simulink model "D53_LKAS_JLU_20200908_1055"  (R2018b)
settings: Solver=ode3  StartTime=0.0  StopTime=10.0  FixedStep=0.01  RelTol=1e-3  EnableMultiTasking=on
model workspace (MAT data in the model file):
  LKA_CarWidth = Simulink.Parameter
  LKA_CarWidth.Value = 1.8
  LKA_CarWidth.DataType = 'single'
  LKA_CarWidth.Dimensions = [1 1]
  LKA_SampleTime = Simulink.Parameter
  LKA_SampleTime.Value = 0.01
  LKA_SampleTime.DataType = 'single'
  LKA_SampleTime.Dimensions = [1 1]
  LKA_StrRatio_C = Simulink.Parameter
  LKA_StrRatio_C.Value = 15.3
  LKA_StrRatio_C.DataType = 'single'
  LKA_StrRatio_C.Dimensions = [1 1]
  LKA_Veh2CamL_C = Simulink.Parameter
  LKA_Veh2CamL_C.Value = 1.56
  LKA_Veh2CamL_C.DataType = 'single'
  LKA_Veh2CamL_C.Dimensions = [1 1]
  LKA_Veh2CamW_C = Simulink.Parameter
  LKA_Veh2CamW_C.Value = 0.9
  LKA_Veh2CamW_C.DataType = 'single'
  LKA_Veh2CamW_C.Dimensions = [1 1]
  LKA_WhlBaseL_C = Simulink.Parameter
  LKA_WhlBaseL_C.Value = 2.65
  LKA_WhlBaseL_C.DataType = 'single'
  LKA_WhlBaseL_C.Dimensions = [1 1]
  LL_CompSWA_C = Simulink.Parameter
  LL_CompSWA_C.Value = 0
  LL_CompSWA_C.DataType = 'single'
  LL_CompSWA_C.Dimensions = [1 1]
  LL_CrvtPrvwT_C = Simulink.Parameter
  LL_CrvtPrvwT_C.Value = 0.45
  LL_CrvtPrvwT_C.DataType = 'single'
  LL_CrvtPrvwT_C.Dimensions = [1 1]
  LL_DesDvt_C = Simulink.Parameter
  LL_DesDvt_C.Value = 0.2
  LL_DesDvt_C.DataType = 'single'
  LL_DesDvt_C.Dimensions = [1 1]
  LL_DvtComp_C = Simulink.Parameter
  LL_DvtComp_C.Value = 0
  LL_DvtComp_C.DataType = 'single'
  LL_DvtComp_C.Dimensions = [1 1]
  LL_DvtPrvwT_C = Simulink.Parameter
  LL_DvtPrvwT_C.Value = 0.45
  LL_DvtPrvwT_C.DataType = 'single'
  LL_DvtPrvwT_C.Dimensions = [1 1]
  LL_DvtSpdDet_vDvtSpdMin_C = Simulink.Parameter
  LL_DvtSpdDet_vDvtSpdMin_C.Value = 0
  LL_DvtSpdDet_vDvtSpdMin_C.DataType = 'single'
  LL_DvtSpdDet_vDvtSpdMin_C.Dimensions = [1 1]
  LL_HdAgExT_C = Simulink.Parameter
  LL_HdAgExT_C.Value = 15
  LL_HdAgExT_C.DataType = 'single'
  LL_HdAgExT_C.Dimensions = [1 1]
  LL_HdAgPrvwT_C = Simulink.Parameter
  LL_HdAgPrvwT_C.Value = 0.45
  LL_HdAgPrvwT_C.DataType = 'single'
  LL_HdAgPrvwT_C.Dimensions = [1 1]
  LL_LAccMax_C = Simulink.Parameter
  LL_LAccMax_C.Value = 3
  LL_LAccMax_C.DataType = 'single'
  LL_LAccMax_C.Dimensions = [1 1]
  LL_LAccRMax_C = Simulink.Parameter
  LL_LAccRMax_C.Value = 5
  LL_LAccRMax_C.DataType = 'single'
  LL_LAccRMax_C.Dimensions = [1 1]
  LL_LDWS_SUPPRESS_HEADING = Simulink.Parameter
  LL_LDWS_SUPPRESS_HEADING.Value = 2
  LL_LDWS_SUPPRESS_HEADING.DataType = 'single'
  LL_LDWS_SUPPRESS_HEADING.Dimensions = [1 1]
  LL_LDW_EarliestWarnLine_C = Simulink.Parameter
  LL_LDW_EarliestWarnLine_C.Value = 0.3
  LL_LDW_EarliestWarnLine_C.DataType = 'single'
  LL_LDW_EarliestWarnLine_C.Dimensions = [1 1]
  LL_LDW_LatestWarnLine_C = Simulink.Parameter
  LL_LDW_LatestWarnLine_C.Value = -0.4
  LL_LDW_LatestWarnLine_C.DataType = 'single'
  LL_LDW_LatestWarnLine_C.Dimensions = [1 1]
  LL_LFClb_TFC_DiffCtlBalance = Simulink.Parameter
  LL_LFClb_TFC_DiffCtlBalance.Value = 0
  LL_LFClb_TFC_DiffCtlBalance.DataType = 'single'
  LL_LFClb_TFC_DiffCtlBalance.Dimensions = [1 1]
  LL_LFClb_TFC_DiffCtrlMaxSWA = Simulink.Parameter
  LL_LFClb_TFC_DiffCtrlMaxSWA.Value = 20
  LL_LFClb_TFC_DiffCtrlMaxSWA.DataType = 'single'
  LL_LFClb_TFC_DiffCtrlMaxSWA.Dimensions = [1 1]
  LL_LFClb_TFC_DiffCtrlRatio = Simulink.Parameter
  LL_LFClb_TFC_DiffCtrlRatio.Value = 400
  LL_LFClb_TFC_DiffCtrlRatio.DataType = 'single'
  LL_LFClb_TFC_DiffCtrlRatio.Dimensions = [1 1]
  LL_LFClb_TFC_FfCtlRatio_C = Simulink.Parameter
  LL_LFClb_TFC_FfCtlRatio_C.Value = 1
  LL_LFClb_TFC_FfCtlRatio_C.DataType = 'single'
  LL_LFClb_TFC_FfCtlRatio_C.Dimensions = [1 1]
  LL_LFClb_TFC_facmGainLutGain1_C = Simulink.Parameter
  LL_LFClb_TFC_facmGainLutGain1_C.Value = 40
  LL_LFClb_TFC_facmGainLutGain1_C.DataType = 'single'
  LL_LFClb_TFC_facmGainLutGain1_C.Dimensions = [1 1]
  LL_LFClb_TFC_facmGainLutGain2_C = Simulink.Parameter
  LL_LFClb_TFC_facmGainLutGain2_C.Value = 40
  LL_LFClb_TFC_facmGainLutGain2_C.DataType = 'single'
  LL_LFClb_TFC_facmGainLutGain2_C.Dimensions = [1 1]
  LL_LFClb_TFC_facmIntegRatio = Simulink.Parameter
  LL_LFClb_TFC_facmIntegRatio.Value = 0.002
  LL_LFClb_TFC_facmIntegRatio.DataType = 'single'
  LL_LFClb_TFC_facmIntegRatio.Dimensions = [1 1]
  LL_LFClb_TFC_facmKlat_C = Simulink.Parameter
  LL_LFClb_TFC_facmKlat_C.Value = -9
  LL_LFClb_TFC_facmKlat_C.DataType = 'single'
  LL_LFClb_TFC_facmKlat_C.Dimensions = [1 1]
  LL_LFClb_TFC_phiIntegCtlMaxSWA_C = Simulink.Parameter
  LL_LFClb_TFC_phiIntegCtlMaxSWA_C.Value = 5
  LL_LFClb_TFC_phiIntegCtlMaxSWA_C.DataType = 'single'
  LL_LFClb_TFC_phiIntegCtlMaxSWA_C.Dimensions = [1 1]
  LL_LFClb_TFC_tiKlatPrvwT_C = Simulink.Parameter
  LL_LFClb_TFC_tiKlatPrvwT_C.Value = 2
  LL_LFClb_TFC_tiKlatPrvwT_C.DataType = 'single'
  LL_LFClb_TFC_tiKlatPrvwT_C.Dimensions = [1 1]
  LL_LFClb_TFC_vGainLutVehSpdLwr_C = Simulink.Parameter
  LL_LFClb_TFC_vGainLutVehSpdLwr_C.Value = 60
  LL_LFClb_TFC_vGainLutVehSpdLwr_C.DataType = 'single'
  LL_LFClb_TFC_vGainLutVehSpdLwr_C.Dimensions = [1 1]
  LL_LFClb_TFC_vGainLutVehSpdUpr_C = Simulink.Parameter
  LL_LFClb_TFC_vGainLutVehSpdUpr_C.Value = 120
  LL_LFClb_TFC_vGainLutVehSpdUpr_C.DataType = 'single'
  LL_LFClb_TFC_vGainLutVehSpdUpr_C.Dimensions = [1 1]
  LL_LKAExPrcs_ExitC0Dvt = Simulink.Parameter
  LL_LKAExPrcs_ExitC0Dvt.Value = 0.01
  LL_LKAExPrcs_ExitC0Dvt.DataType = 'single'
  LL_LKAExPrcs_ExitC0Dvt.Dimensions = [1 1]
  LL_LKAExPrcs_ExitC0Swt = Simulink.Parameter
  LL_LKAExPrcs_ExitC0Swt.Value = 1
  LL_LKAExPrcs_ExitC0Swt.DataType = 'single'
  LL_LKAExPrcs_ExitC0Swt.Dimensions = [1 1]
  LL_LKAExPrcs_tiExitTime1 = Simulink.Parameter
  LL_LKAExPrcs_tiExitTime1.Value = 8
  LL_LKAExPrcs_tiExitTime1.DataType = 'single'
  LL_LKAExPrcs_tiExitTime1.Dimensions = [1 1]
  LL_LKAExPrcs_tiExitTime2 = Simulink.Parameter
  LL_LKAExPrcs_tiExitTime2.Value = 4
  LL_LKAExPrcs_tiExitTime2.DataType = 'single'
  LL_LKAExPrcs_tiExitTime2.Dimensions = [1 1]
  LL_LKAExPrcs_tiExitTime3 = Simulink.Parameter
  LL_LKAExPrcs_tiExitTime3.Value = 0.2
  LL_LKAExPrcs_tiExitTime3.DataType = 'single'
  LL_LKAExPrcs_tiExitTime3.Dimensions = [1 1]
  LL_LKASWASyn_M0 = Simulink.Parameter
  LL_LKASWASyn_M0.Value = 0.4
  LL_LKASWASyn_M0.DataType = 'single'
  LL_LKASWASyn_M0.Dimensions = [1 1]
  LL_LKASWASyn_M1 = Simulink.Parameter
  LL_LKASWASyn_M1.Value = 0.8
  LL_LKASWASyn_M1.DataType = 'single'
  LL_LKASWASyn_M1.Dimensions = [1 1]
  LL_LKASWASyn_M2 = Simulink.Parameter
  LL_LKASWASyn_M2.Value = 0.3
  LL_LKASWASyn_M2.DataType = 'single'
  LL_LKASWASyn_M2.Dimensions = [1 1]
  LL_LKASWASyn_M3K = Simulink.Parameter
  LL_LKASWASyn_M3K.Value = 0.2
  LL_LKASWASyn_M3K.DataType = 'single'
  LL_LKASWASyn_M3K.Dimensions = [1 1]
  LL_LKASWASyn_SWAaddMax = Simulink.Parameter
  LL_LKASWASyn_SWAaddMax.Value = 8
  LL_LKASWASyn_SWAaddMax.DataType = 'single'
  LL_LKASWASyn_SWAaddMax.Dimensions = [1 1]
  LL_LKASWASyn_T2 = Simulink.Parameter
  LL_LKASWASyn_T2.Value = 4
  LL_LKASWASyn_T2.DataType = 'single'
  LL_LKASWASyn_T2.Dimensions = [1 1]
  LL_LKASWASyn_TrqMax = Simulink.Parameter
  LL_LKASWASyn_TrqMax.Value = 1.5
  LL_LKASWASyn_TrqMax.DataType = 'single'
  LL_LKASWASyn_TrqMax.Dimensions = [1 1]
  LL_LKASWASyn_TrqSwaAddSwt = Simulink.Parameter
  LL_LKASWASyn_TrqSwaAddSwt.Value = 0
  LL_LKASWASyn_TrqSwaAddSwt.DataType = 'single'
  LL_LKASWASyn_TrqSwaAddSwt.Dimensions = [1 1]
  LL_LKASWASyn_TrqSwaRateDiff = Simulink.Parameter
  LL_LKASWASyn_TrqSwaRateDiff.Value = -0.2
  LL_LKASWASyn_TrqSwaRateDiff.DataType = 'single'
  LL_LKASWASyn_TrqSwaRateDiff.Dimensions = [1 1]
  LL_LKASWASyn_tiTrqSwaRtTime = Simulink.Parameter
  LL_LKASWASyn_tiTrqSwaRtTime.Value = 0.2
  LL_LKASWASyn_tiTrqSwaRtTime.DataType = 'single'
  LL_LKASWASyn_tiTrqSwaRtTime.Dimensions = [1 1]
  LL_LKASWASyn_tiTrqSwaTime = Simulink.Parameter
  LL_LKASWASyn_tiTrqSwaTime.Value = 0.3
  LL_LKASWASyn_tiTrqSwaTime.DataType = 'single'
  LL_LKASWASyn_tiTrqSwaTime.Dimensions = [1 1]
  LL_LKAS_OUT_OF_CONTROL_LAT_VEL = Simulink.Parameter
  LL_LKAS_OUT_OF_CONTROL_LAT_VEL.Value = 1.5
  LL_LKAS_OUT_OF_CONTROL_LAT_VEL.DataType = 'single'
  LL_LKAS_OUT_OF_CONTROL_LAT_VEL.Dimensions = [1 1]
  LL_LKAS_OUT_OF_CONTROL_TTLC = Simulink.Parameter
  LL_LKAS_OUT_OF_CONTROL_TTLC.Value = 0.3
  LL_LKAS_OUT_OF_CONTROL_TTLC.DataType = 'single'
  LL_LKAS_OUT_OF_CONTROL_TTLC.Dimensions = [1 1]
  LL_LKA_EarliestWarnLine_C = Simulink.Parameter
  LL_LKA_EarliestWarnLine_C.Value = 0.3
  LL_LKA_EarliestWarnLine_C.DataType = 'single'
  LL_LKA_EarliestWarnLine_C.Dimensions = [1 1]
  LL_LKA_LatestWarnLine_C = Simulink.Parameter
  LL_LKA_LatestWarnLine_C.Value = -0.5
  LL_LKA_LatestWarnLine_C.DataType = 'single'
  LL_LKA_LatestWarnLine_C.Dimensions = [1 1]
  LL_LSpdCompT_C = Simulink.Parameter
  LL_LSpdCompT_C.Value = 0.4
  LL_LSpdCompT_C.DataType = 'single'
  LL_LSpdCompT_C.Dimensions = [1 1]
  LL_MAX_DELAY_EPSSTAR_TIME = Simulink.Parameter
  LL_MAX_DELAY_EPSSTAR_TIME.Value = 0.5
  LL_MAX_DELAY_EPSSTAR_TIME.DataType = 'single'
  LL_MAX_DELAY_EPSSTAR_TIME.Dimensions = [1 1]
  LL_MAX_DRIVER_TORQUE_DISABLE = Simulink.Parameter
  LL_MAX_DRIVER_TORQUE_DISABLE.Value = 2.25
  LL_MAX_DRIVER_TORQUE_DISABLE.DataType = 'single'
  LL_MAX_DRIVER_TORQUE_DISABLE.Dimensions = [1 1]
  LL_MAX_DRIVER_TORQUE_ENABLE = Simulink.Parameter
  LL_MAX_DRIVER_TORQUE_ENABLE.Value = 3
  LL_MAX_DRIVER_TORQUE_ENABLE.DataType = 'single'
  LL_MAX_DRIVER_TORQUE_ENABLE.Dimensions = [1 1]
  LL_MAX_LANE_WIDTH_DISABLE = Simulink.Parameter
  LL_MAX_LANE_WIDTH_DISABLE.Value = 5.5
  LL_MAX_LANE_WIDTH_DISABLE.DataType = 'single'
  LL_MAX_LANE_WIDTH_DISABLE.Dimensions = [1 1]
  LL_MAX_LANE_WIDTH_ENABLE = Simulink.Parameter
  LL_MAX_LANE_WIDTH_ENABLE.Value = 5.4
  LL_MAX_LANE_WIDTH_ENABLE.DataType = 'single'
  LL_MAX_LANE_WIDTH_ENABLE.Dimensions = [1 1]
  LL_MAX_LAT_ACC_DISABLE = Simulink.Parameter
  LL_MAX_LAT_ACC_DISABLE.Value = 3.5
  LL_MAX_LAT_ACC_DISABLE.DataType = 'single'
  LL_MAX_LAT_ACC_DISABLE.Dimensions = [1 1]
  LL_MAX_LAT_ACC_ENABLE = Simulink.Parameter
  LL_MAX_LAT_ACC_ENABLE.Value = 3
  LL_MAX_LAT_ACC_ENABLE.DataType = 'single'
  LL_MAX_LAT_ACC_ENABLE.Dimensions = [1 1]
  LL_MAX_LDWS_SPEED_DISABLE = Simulink.Parameter
  LL_MAX_LDWS_SPEED_DISABLE.Value = 150
  LL_MAX_LDWS_SPEED_DISABLE.DataType = 'single'
  LL_MAX_LDWS_SPEED_DISABLE.Dimensions = [1 1]
  LL_MAX_LDWS_SPEED_ENABLE = Simulink.Parameter
  LL_MAX_LDWS_SPEED_ENABLE.Value = 140
  LL_MAX_LDWS_SPEED_ENABLE.DataType = 'single'
  LL_MAX_LDWS_SPEED_ENABLE.Dimensions = [1 1]
  LL_MAX_LKAS_SPEED_DISABLE = Simulink.Parameter
  LL_MAX_LKAS_SPEED_DISABLE.Value = 150
  LL_MAX_LKAS_SPEED_DISABLE.DataType = 'single'
  LL_MAX_LKAS_SPEED_DISABLE.Dimensions = [1 1]
  LL_MAX_LKAS_SPEED_ENABLE = Simulink.Parameter
  LL_MAX_LKAS_SPEED_ENABLE.Value = 140
  LL_MAX_LKAS_SPEED_ENABLE.DataType = 'single'
  LL_MAX_LKAS_SPEED_ENABLE.Dimensions = [1 1]
  LL_MAX_LONG_ACC_DISABLE = Simulink.Parameter
  LL_MAX_LONG_ACC_DISABLE.Value = 3.5
  LL_MAX_LONG_ACC_DISABLE.DataType = 'single'
  LL_MAX_LONG_ACC_DISABLE.Dimensions = [1 1]
  LL_MAX_LONG_ACC_ENABLE = Simulink.Parameter
  LL_MAX_LONG_ACC_ENABLE.Value = 3
  LL_MAX_LONG_ACC_ENABLE.DataType = 'single'
  LL_MAX_LONG_ACC_ENABLE.Dimensions = [1 1]
  LL_MAX_LONG_DECEL_DISABLE = Simulink.Parameter
  LL_MAX_LONG_DECEL_DISABLE.Value = 2.5
  LL_MAX_LONG_DECEL_DISABLE.DataType = 'single'
  LL_MAX_LONG_DECEL_DISABLE.Dimensions = [1 1]
  LL_MAX_LONG_DECEL_ENABLE = Simulink.Parameter
  LL_MAX_LONG_DECEL_ENABLE.Value = 2
  LL_MAX_LONG_DECEL_ENABLE.DataType = 'single'
  LL_MAX_LONG_DECEL_ENABLE.Dimensions = [1 1]
  LL_MAX_STEER_ANGLE_DISABLE = Simulink.Parameter
  LL_MAX_STEER_ANGLE_DISABLE.Value = 70
  LL_MAX_STEER_ANGLE_DISABLE.DataType = 'single'
  LL_MAX_STEER_ANGLE_DISABLE.Dimensions = [1 1]
  LL_MAX_STEER_ANGLE_ENABLE = Simulink.Parameter
  LL_MAX_STEER_ANGLE_ENABLE.Value = 60
  LL_MAX_STEER_ANGLE_ENABLE.DataType = 'single'
  LL_MAX_STEER_ANGLE_ENABLE.Dimensions = [1 1]
  LL_MAX_STEER_SPEED_DISABLE = Simulink.Parameter
  LL_MAX_STEER_SPEED_DISABLE.Value = 5000
  LL_MAX_STEER_SPEED_DISABLE.DataType = 'single'
  LL_MAX_STEER_SPEED_DISABLE.Dimensions = [1 1]
  LL_MAX_STEER_SPEED_ENABLE = Simulink.Parameter
  LL_MAX_STEER_SPEED_ENABLE.Value = 5000
  LL_MAX_STEER_SPEED_ENABLE.DataType = 'single'
  LL_MAX_STEER_SPEED_ENABLE.Dimensions = [1 1]
  LL_MAX_SYSTEM_CURVATURE_DISABLE = Simulink.Parameter
  LL_MAX_SYSTEM_CURVATURE_DISABLE.Value = 0.0055
  LL_MAX_SYSTEM_CURVATURE_DISABLE.DataType = 'single'
  LL_MAX_SYSTEM_CURVATURE_DISABLE.Dimensions = [1 1]
  LL_MAX_SYSTEM_CURVATURE_ENABLE = Simulink.Parameter
  LL_MAX_SYSTEM_CURVATURE_ENABLE.Value = 0.0045
  LL_MAX_SYSTEM_CURVATURE_ENABLE.DataType = 'single'
  LL_MAX_SYSTEM_CURVATURE_ENABLE.Dimensions = [1 1]
  LL_MIN_LANE_WIDTH_DISABLE = Simulink.Parameter
  LL_MIN_LANE_WIDTH_DISABLE.Value = 2.4
  LL_MIN_LANE_WIDTH_DISABLE.DataType = 'single'
  LL_MIN_LANE_WIDTH_DISABLE.Dimensions = [1 1]
  LL_MIN_LANE_WIDTH_ENABLE = Simulink.Parameter
  LL_MIN_LANE_WIDTH_ENABLE.Value = 2.5
  LL_MIN_LANE_WIDTH_ENABLE.DataType = 'single'
  LL_MIN_LANE_WIDTH_ENABLE.Dimensions = [1 1]
  LL_MIN_LKAS_SPEED_DISABLE = Simulink.Parameter
  LL_MIN_LKAS_SPEED_DISABLE.Value = 55
  LL_MIN_LKAS_SPEED_DISABLE.DataType = 'single'
  LL_MIN_LKAS_SPEED_DISABLE.Dimensions = [1 1]
  LL_MIN_LKAS_SPEED_ENABLE = Simulink.Parameter
  LL_MIN_LKAS_SPEED_ENABLE.Value = 60
  LL_MIN_LKAS_SPEED_ENABLE.DataType = 'single'
  LL_MIN_LKAS_SPEED_ENABLE.Dimensions = [1 1]
  LL_Max_LDWS_Warning_Time = Simulink.Parameter
  LL_Max_LDWS_Warning_Time.Value = 5
  LL_Max_LDWS_Warning_Time.DataType = 'single'
  LL_Max_LDWS_Warning_Time.Dimensions = [1 1]
  LL_NomTAhd_C = Simulink.Parameter
  LL_NomTAhd_C.Value = 0.2
  LL_NomTAhd_C.DataType = 'single'
  LL_NomTAhd_C.Dimensions = [1 1]
  LL_ThresDet_lDvtThresLwrLDW = Simulink.Parameter
  LL_ThresDet_lDvtThresLwrLDW.Value = 0.15
  LL_ThresDet_lDvtThresLwrLDW.DataType = 'single'
  LL_ThresDet_lDvtThresLwrLDW.Dimensions = [1 1]
  LL_ThresDet_lDvtThresLwrLKA = Simulink.Parameter
  LL_ThresDet_lDvtThresLwrLKA.Value = 0.3
  LL_ThresDet_lDvtThresLwrLKA.DataType = 'single'
  LL_ThresDet_lDvtThresLwrLKA.Dimensions = [1 1]
  LL_ThresDet_lDvtThresUprLDW = Simulink.Parameter
  LL_ThresDet_lDvtThresUprLDW.Value = 0.3
  LL_ThresDet_lDvtThresUprLDW.DataType = 'single'
  LL_ThresDet_lDvtThresUprLDW.Dimensions = [1 1]
  LL_ThresDet_lDvtThresUprLKA = Simulink.Parameter
  LL_ThresDet_lDvtThresUprLKA.Value = 0.6
  LL_ThresDet_lDvtThresUprLKA.DataType = 'single'
  LL_ThresDet_lDvtThresUprLKA.Dimensions = [1 1]
  LL_ThresDet_tiTTLCThresLDW = Simulink.Parameter
  LL_ThresDet_tiTTLCThresLDW.Value = 0.75
  LL_ThresDet_tiTTLCThresLDW.DataType = 'single'
  LL_ThresDet_tiTTLCThresLDW.Dimensions = [1 1]
  LL_ThresDet_tiTTLCThresLKA = Simulink.Parameter
  LL_ThresDet_tiTTLCThresLKA.Value = 1.5
  LL_ThresDet_tiTTLCThresLKA.DataType = 'single'
  LL_ThresDet_tiTTLCThresLKA.Dimensions = [1 1]
  LL_TkOvStChk_tiTDelTime = Simulink.Parameter
  LL_TkOvStChk_tiTDelTime.Value = 2
  LL_TkOvStChk_tiTDelTime.DataType = 'single'
  LL_TkOvStChk_tiTDelTime.Dimensions = [1 1]
  LL_TkOvStChk_tiTrqChkT = Simulink.Parameter
  LL_TkOvStChk_tiTrqChkT.Value = 0.1
  LL_TkOvStChk_tiTrqChkT.DataType = 'single'
  LL_TkOvStChk_tiTrqChkT.Dimensions = [1 1]
  LL_lStpLngth_C = Simulink.Parameter
  LL_lStpLngth_C.Value = 5
  LL_lStpLngth_C.DataType = 'single'
  LL_lStpLngth_C.Dimensions = [1 1]
  ob_LKA_Version = Simulink.Signal
  ob_LKA_Version.DataType = 'single'
  ob_LKA_Version.Dimensions = -1
  ob_LKA_Version.DimensionsMode = 'auto'
  ob_LKA_Version.Complexity = 'auto'
  ob_LKA_Version.SampleTime = -1
  ob_LKA_Version.SamplingMode = 'auto'
undefined symbols (not defined in the file): LKA_CarWidth, LKA_SampleTime, LKA_StrRatio_C, LKA_Veh2CamL_C, LKA_Veh2CamW_C, LKA_WhlBaseL_C, LL_CompSWA_C, LL_CrvtPrvwT_C, LL_DesDvt_C, LL_DvtComp_C, LL_DvtPrvwT_C, LL_DvtSpdDet_vDvtSpdMin_C, LL_HdAgExT_C, LL_HdAgPrvwT_C, LL_LAccMax_C, LL_LAccRMax_C, LL_LDW_EarliestWarnLine_C, LL_LDW_LatestWarnLine_C, LL_LDWS_SUPPRESS_HEADING, LL_LFClb_TFC_DiffCtlBalance, LL_LFClb_TFC_DiffCtrlMaxSWA, LL_LFClb_TFC_DiffCtrlRatio, LL_LFClb_TFC_facmGainLutGain1_C, LL_LFClb_TFC_facmGainLutGain2_C, LL_LFClb_TFC_facmIntegRatio, LL_LFClb_TFC_facmKlat_C, LL_LFClb_TFC_FfCtlRatio_C, LL_LFClb_TFC_phiIntegCtlMaxSWA_C, LL_LFClb_TFC_tiKlatPrvwT_C, LL_LFClb_TFC_vGainLutVehSpdLwr_C, LL_LFClb_TFC_vGainLutVehSpdUpr_C, LL_LKA_EarliestWarnLine_C, LL_LKA_LatestWarnLine_C, LL_LKAExPrcs_ExitC0Dvt, LL_LKAExPrcs_ExitC0Swt, LL_LKAExPrcs_tiExitTime1, LL_LKAExPrcs_tiExitTime2, LL_LKAExPrcs_tiExitTime3, LL_LKAS_OUT_OF_CONTROL_LAT_VEL, LL_LKAS_OUT_OF_CONTROL_TTLC, LL_LKASWASyn_M0, LL_LKASWASyn_M1, LL_LKASWASyn_M2, LL_LKASWASyn_M3K, LL_LKASWASyn_SWAaddMax, LL_LKASWASyn_T2, LL_LKASWASyn_tiTrqSwaRtTime, LL_LKASWASyn_tiTrqSwaTime, LL_LKASWASyn_TrqMax, LL_LKASWASyn_TrqSwaAddSwt, LL_LKASWASyn_TrqSwaRateDiff, LL_LSpdCompT_C, LL_lStpLngth_C, LL_MAX_DELAY_EPSSTAR_TIME, LL_MAX_DRIVER_TORQUE_DISABLE, LL_MAX_DRIVER_TORQUE_ENABLE, LL_MAX_LANE_WIDTH_DISABLE, LL_MAX_LANE_WIDTH_ENABLE, LL_MAX_LAT_ACC_DISABLE, LL_MAX_LAT_ACC_ENABLE ... (+30)
libraries: simulink x134, canmsglib x36, dspstat3 x3, simulink_extras x1
(part 1 of 17)
settings Model: Creator=Administrator  LastModifiedBy=ADMIN
settings DataIOCC: LimitDataPoints=on  SaveFormat=Array
settings OptimizationCC: LifeSpan=1
settings DebuggingCC: UnderspecifiedInitializationDetection=Classic  MergeDetectMultiDrivingBlocksExec=none  SolverPrmCheckMsg=warning  MultiTaskDSMMsg=warning  SFUnexpectedBacktrackingDiag=warning  SFNoUnconditionalDefaultTransitionDiag=warning  SFExecutionAtInitializationDiag=none
settings HardwareCC: ProdBitPerPointer=32  ProdBitPerSizeT=32  ProdBitPerPtrDiffT=32  ProdLargestAtomicInteger=Long  ProdLargestAtomicFloat=Double  ProdEndianess=BigEndian  ProdWordSize=32  ProdHWDeviceType=Freescale->MPC5xx
settings ModelReferenceCC: PropagateSignalLabelsOutOfModel=off
settings SFSimCC: SimUseLocalCustomCode=off  MATLABDynamicMemAlloc=off
settings RTWCC: SystemTargetFile=hc12.tlc  GenerateMakefile=off  TemplateMakefile=hc12_default_tmf  Description=Embedded Target for Motorola HC12 and CodeWarrior (real-time)  RTWUseLocalCustomCode=off
settings CodeAppCC: IgnoreCustomStorageClasses=off  StateflowObjectComments=on
settings STFCustomTargetCC: TargetLangStandard=C99 (ISO)  CodeReplacementLibrary=C89/C90 (ANSI)  ModelReferenceCompliant=off  CombineOutputUpdateFcns=on  ERTCustomFileBanners=on  SupportContinuousTime=off  SupportNonInlinedSFcns=off  RemoveResetFunc=on  MATLABClassNameForMDSCustomization=Simulink.SoftwareTarget.ERTCustomization  SystemTargetFile=hc12.tlc
settings ERTTargetCC: TargetLangStandard=C99 (ISO)  CodeReplacementLibrary=C89/C90 (ANSI)  MultiwordLength=2048  ModelReferenceCompliant=off  ParMdlRefBuildCompliant=off  CompOptLevelCompliant=off  ConcurrentExecutionCompliant=off  ModelStepFunctionPrototypeControlCompliant=off  CPPClassGenCompliant=off  UseToolchainInfoCompliant=off  ERTCustomFileTemplate=hc12_file_process.tlc  ConvertIfToSwitch=off  SuppressUnreachableDefaultCases=off
settings ConfigComp: CovMetricSettings=dw  CovHtmlReporting=on  CovSaveCumulativeToWorkspaceVar=on  CovSaveSingleToWorkspaceVar=on  CovExternalEMLEnable=off

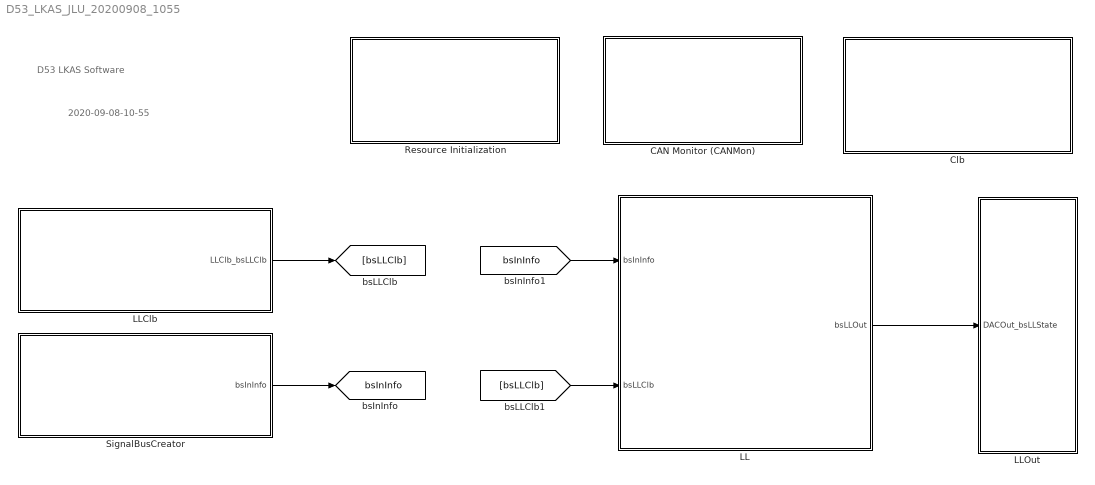
== system D53_LKAS_JLU_20200908_1055 ==
  note: D53 LKAS Software
  note: 2020-09-08-10-55
  CAN Monitor (CANMon) : Subsystem
      mask Display:
      | color('blue');
      | text(0.98,0.9,'iPilot Software Model','horizontalAlignment','right');
      | color('black');
      | text(0.5,0.5,'CAN Monintor(CANMon)','horizontalAlignment','center');
      | text(0.5,0.4,'(10ms)','horizontalAlignment','center');
  Clb : Subsystem
  LL : Subsystem
  LLClb : Subsystem
  LLOut : Subsystem
  Resource Initialization : Subsystem
      mask Display:
      | color('green');
      | text(0.98,0.9,'iPilot Control Software Model','horizontalAlignment','right');
      | color('green');
      | text(0.5,0.5,'Resource Initialization','horizontalAlignment','center');
  SignalBusCreator : Subsystem
  tag scope: bsInInfo=global
  wires:
  SignalBusCreator/1(bsInInfo) -> [bsInInfo]
  LLClb/1(LLClb_bsLLClb) -> [bsLLClb]
  [bsInInfo] -> LL/1(bsInInfo)
  [bsLLClb] -> LL/2(bsLLClb)
  LL/1(bsLLOut) -> LLOut/1(DACOut_bsLLState)

== system D53_LKAS_JLU_20200908_1055/CAN Monitor (CANMon) ==
  Input : Subsystem  Commented=on
  Monitor : Subsystem
  Output : Subsystem  Commented=on

== system D53_LKAS_JLU_20200908_1055/Clb ==
  CAN Unpack : canmsglib/CAN Unpack  Commented=on  MsgList=(none)  MsgName=CAN Msg  MsgIDType=Extended (29-bit identifier)  MsgIdentifier=120534787  MsgLength=8  SignalInfo=Serial number$0$8$1$2$1$0$1$0$-Inf$Inf$#index$8$8$1$2$1$0$1$-100$-Inf$Inf$#coefficient$16$32$1$2$1$0$0.000001$-10$-Inf$Inf$#  NSignals=3  IDPort=off  TimestampPort=off  ErrorPort=off  RemotePort=off  LengthPort=off  StatusPort=off  StartBits=str2num('[int32(0);int32(8);int32(16)]')  SignalSizes=str2num('[int32(8);int32(8);int32(32)]')  ByteOrders=str2num('[int32(1);int32(1);int32(1)]')  DataTypes=str2num('[int32(2);int32(2);int32(2)]')  MultiplexTypes=str2num('[int32(1);int32(1);int32(1)]')  MultiplexValues=str2num('[double(0);double(0);double(0)]')  Factors=str2num('[double(1);double(1);double(0.000001)]')  Offsets=str2num('[double(0);double(-100);double(-10)]')  Minimums=str2num('[double(-Inf);double(-Inf);double(-Inf)]')  Maximums=str2num('[double(Inf);double(Inf);double(Inf)]')  ApplyMinMax=off
      settings: SourceProductName=Simulink Real-Time  SourceProductBaseCode=XP
  Calibration1 : Subsystem
  Calibration2 : Subsystem
  Calibration3 : Subsystem
  S-Function2 : S-Function  Commented=on  FunctionName=CAN_Rec_P  Parameters=uint8(Module-1),uint32(ID),uint8(Frameformat-1),uint8(Newflag),uint8(FIFO),double(sampletime)  SFunctionDeploymentMode=off  EnableBusSupport=off  mask(CAN_receive){Module=CAN_0, ID=256, Frameformat=Extended (29-bit identifier), Newflag=on, FIFO=off, sampletime=0.01}
      mask prompts: Module "CAN Port:"; ID "CAN Frame ID:"; Frameformat "CAN Frame Format:"; FIFO "Overflow flag"
      mask init:
      | maskdisplay = canrecicon(Module,ID,Frameformat,Newflag,FIFO);
      | set_param(gcb, 'MaskDisplay', maskdisplay);
      mask TypeOptions Module: CAN_0 | CAN_1 | CAN_2 | CAN_3
      mask TypeOptions Frameformat: Standard (11-bit identifier) | Extended (29-bit identifier)
      mask Display: color('blue');text(0.98,0.9,'MPC5675K','horizontalAlignment','right');color('black');text(0.5,0.6,'FlexCAN_0 Receive','horizontalAlignment','center');text(0.5,0.35,'Extended ID:256','horizontalAlignment','center');port_label('output',1,'New_Flag');port_label('output',2,'CAN_Msg');
  Subsystem1 : Subsystem
  Subsystem5 : Subsystem
  tag scope: LL_LKASWASyn_M0=global, LL_LKASWASyn_M1=global, LL_LKASWASyn_M2=global, LL_LKASWASyn_M3K=global, LL_LKASWASyn_T2=global, LL_MIN_LKAS_SPEED_DISABLE=global, LL_MIN_LKAS_SPEED_ENABLE=global, empty10=global, empty11=global, empty12=global, empty13=global, empty14=global, empty15=global, empty16=global, empty17=global, empty18=global, empty19=global, empty20=global, empty21=global, empty22=global, empty23=global, empty24=global, empty25=global, empty26=global, empty27=global, empty28=global, empty29=global, empty30=global, empty8=global, empty9=global
  wires:
  Subsystem1/2(Out2) -> Subsystem5/1(In1)
  Subsystem1/3(Out3) -> Subsystem5/2(In2)
  Subsystem5/1(Out1) -> Calibration3/2(In2), Calibration2/2(In2), Calibration1/2(In2)
  Subsystem1/1(Out1) -> Calibration3/1(In1), Calibration2/1(In1), Calibration1/1(In1)
  S-Function2/2 -> CAN Unpack/1
  Calibration1/1(Out1) -> [LL_LKASWASyn_M0]
  Calibration1/2(Out2) -> [LL_LKASWASyn_M1]
  Calibration1/3(Out3) -> [LL_LKASWASyn_M2]
  Calibration1/4(Out4) -> [LL_LKASWASyn_T2]
  Calibration1/5(Out5) -> [LL_LKASWASyn_M3K]
  Calibration1/6(Out6) -> [LL_MIN_LKAS_SPEED_DISABLE]
  Calibration1/7(Out7) -> [LL_MIN_LKAS_SPEED_ENABLE]
  Calibration1/8(Out8) -> [empty8]
  Calibration1/9(Out9) -> [empty9]
  Calibration1/10(Out10) -> [empty10]
  Calibration2/7(Out7) -> [empty17]
  Calibration2/10(Out10) -> [empty20]
  Calibration2/3(Out3) -> [empty13]
  Calibration2/2(Out2) -> [empty12]
  Calibration2/5(Out5) -> [empty15]
  Calibration2/1(Out1) -> [empty11]
  Calibration2/9(Out9) -> [empty19]
  Calibration2/8(Out8) -> [empty18]
  Calibration2/4(Out4) -> [empty14]
  Calibration2/6(Out6) -> [empty16]
  Calibration3/7(Out7) -> [empty27]
  Calibration3/10(Out10) -> [empty30]
  Calibration3/3(Out3) -> [empty23]
  Calibration3/2(Out2) -> [empty22]
  Calibration3/5(Out5) -> [empty25]
  Calibration3/1(Out1) -> [empty21]
  Calibration3/9(Out9) -> [empty29]
  Calibration3/8(Out8) -> [empty28]
  Calibration3/4(Out4) -> [empty24]
  Calibration3/6(Out6) -> [empty26]

== system D53_LKAS_JLU_20200908_1055/LL ==
  bsInInfo : Inport
  bsLLClb : Inport  Port=2
  Bus Selector1 : BusSelector  OutputSignals=bsLaneInfo.bsR0Info.R0_Q,bsLaneInfo.bsL0Info.L0_Q
  Bus Selector2 : BusSelector  OutputSignals=bsEPSInfo
  Bus Selector3 : BusSelector  OutputSignals=LKA_State,LDW_State
  Bus Selector4 : BusSelector  OutputSignals=bsLaneInfo.Fusion_AdditionalInf.Carema_Status
  Fault_Diagnostic : Subsystem
  Ground1 : Ground
  Ground3 : Ground
  Human Machine Interface (HMI) : Subsystem
  LL Inputs Mapping : Subsystem
  LL Output (LLOut) : Subsystem
  LLOn : Subsystem
  Subsystem : Subsystem
  Terminator : Terminator
  Version : Constant  Value=200428  OutMin=20410  OutMax=200630  OutDataTypeStr=single
  bsLLOut : Outport
  tag scope: LLMon=global
  wires:
  LLOn/5(LLMon) -> [LLMon]
  [bsInInfo] -> Fault_Diagnostic/1(bsInInfo)
  Fault_Diagnostic/1(bsSignalFault) -> [bsSignalFault]
  LLOn/4(M) -> [LLOn_M]
  [bsInfo] -> LLOn/2(bsInInfo)
  [bsSignalFault] -> LLOn/4(bsSignalFault)
  LLOn/3(phiSWACmd) -> [LLOn_phiSWACmd]
  LLOn/1(bsLLState) -> [LLOn_bsLLState]
  [bsLLClb] -> LLOn/3(bsLLClb)
  Subsystem/2(Mode) -> [LLOn_stDACMode], LLOn/1(stDACMode)
  [HMI_bsLLHMI] -> LL Output (LLOut)/3(LLOut_bsLLHMI)
  [LLOn_phiSWACmd] -> LL Output (LLOut)/2(LLOut_phiSWACmd)
  [bsInfo] -> Bus Selector1/1, Bus Selector2/1, Bus Selector4/1
  [bsInfo] -> Subsystem/1(bsInfo)
  Ground1/1 -> Human Machine Interface (HMI)/8(HMI_camera_common_fault)
  Bus Selector4/1 -> Human Machine Interface (HMI)/9(HMI_Front_Camera_Blocked)  "<Carema_Status>"
  [LLOn_M] -> LL Output (LLOut)/4(LLOut_M)
  Bus Selector3/2 -> Human Machine Interface (HMI)/4(HMI_LDW_STATE)  "<LDW_State>"
  bsLLClb/1 -> [bsLLClb]
  [LLOn_bsLLState] -> LL Output (LLOut)/1(LLOut_bsLLState)
  Bus Selector1/1 -> Human Machine Interface (HMI)/5(HMI_R0_Quality)  "<R0_Q>"
  LLOn/2(LDW_Flag) -> [LLOn_bsLDWWarnInfo]
  Bus Selector3/1 -> Human Machine Interface (HMI)/3(HMI_LKA_STATE)  "<LKA_State>"
  Bus Selector1/2 -> Human Machine Interface (HMI)/6(HMI_L0_Quality)  "<L0_Q>"
  [LLOn_stDACMode] -> Human Machine Interface (HMI)/1(HMI_stDACmode)
  LL Inputs Mapping/1(bsInfo) -> [bsInfo]
  [bsInInfo] -> LL Inputs Mapping/1(bsInInfo)
  [LLOn_bsLLState] -> Bus Selector3/1
  Version/1 -> Terminator/1  "ob_LKA_Version"
  LL Output (LLOut)/1(LL_bsLLOut) -> bsLLOut/1  "bsLLOut"
  Subsystem/1(On) -> LLOn/Enable
  Bus Selector2/1 -> Human Machine Interface (HMI)/7(HMI_EPSInfo)  "<bsEPSInfo>"
  [LLOn_bsLDWWarnInfo] -> Human Machine Interface (HMI)/2(HMI_LDWWarn)
  Human Machine Interface (HMI)/1(HMI_LDWLKA) -> [HMI_bsLLHMI]  "bsLLHMI"
  Ground3/1 -> Human Machine Interface (HMI)/10(HMI_stFaultCSyn)
  bsInInfo/1 -> [bsInInfo]

== system D53_LKAS_JLU_20200908_1055/LLClb ==
  Bus Creator : BusCreator  Inputs=4
  ConstantClb : Subsystem
  LDWClb : Subsystem
  LKAClb : Subsystem
  LLSMConClb : Subsystem
  LLClb_bsLLClb : Outport
  wires:
  LKAClb/1(LKAClb) -> Bus Creator/3  "bsLKAClb"
  LDWClb/1(LDWClb) -> Bus Creator/2  "bsLDWClb"
  Bus Creator/1 -> LLClb_bsLLClb/1  "bsLLClb"
  LLSMConClb/1(LLSMConClb) -> Bus Creator/1  "bsLLSMConClb"
  ConstantClb/1(ConstantClb) -> Bus Creator/4  "bsConstantClb"

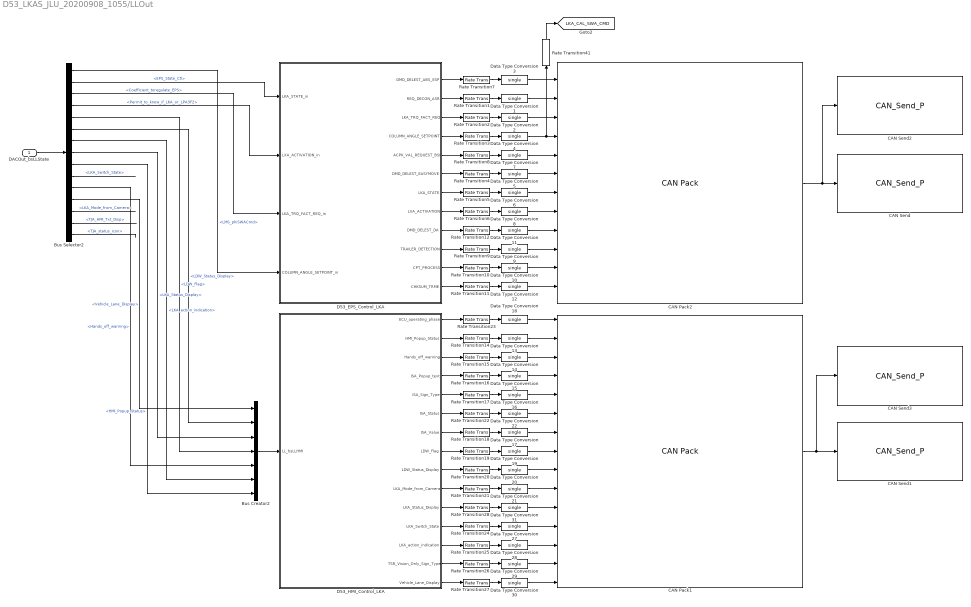
== system D53_LKAS_JLU_20200908_1055/LLOut ==
  DACOut_bsLLState : Inport
  Bus Creator2 : BusCreator  Inputs=7
  Bus Selector2 : BusSelector  OutputSignals=LMS_phiSWACmd,EPS_State_Ctl,Coefficient_toregulate_EPS,Permit_to_know_if_LKA_or_LPA3F2,LDW_Flag,LDW_Status_Display,LKA_action_indication,LKA_Status_Display,HMI_Popup_Status,LKA_Switch_State,Hands_off_warning,Vehicle_Lane_Display,LKA_Mode_from_Camera,TJA_HMI_Txt_Disp,TJA_status_icon
  CAN Pack1 : canmsglib/CAN Pack  CANdbFile=D:\ADAS ECU-PSA1 CAN_for_HIL_20190729_10ms.dbc  MsgList=ADAS_541_PSA1  MsgName=ADAS_541_PSA1  MsgIDType=Standard (11-bit identifier)  MsgIdentifier=1345  MsgLength=8  SignalInfo=ECU_operating_phase$24$4$2$2$1$0$1$0$-Inf$Inf$#HMI_Popup_Status$12$4$2$2$1$0$1$0$-Inf$Inf$#Hands_off_warning$18$1$2$2$1$0$1$0$-Inf$Inf$#ISA_Popup_text$28$3$2$2$1$0$1$0$-Inf$Inf$#ISA_Sign_Type$40$3$2$2$1$0$1$0$-Inf$Inf$#ISA_Status$43$3$2$2$1$0$1$0$-Inf$Inf$#ISA_Value$32$5$2$1$1$0$1$0$0$31$#LDW_Flag$16$2$2$2$1$0$1$0$-Inf$Inf$#LDW_Status_Display$3$2$2$2$1$0$1$0$-Inf$Inf$#LKA_Mode_from_Camera$19$2$2$2$1$0$1$0$-Inf$Inf$#LKA_Status_Display$5$2$2$2$1$0$1$0$-Inf$Inf$#LKA_Switch_State$21$1$2$2$1$0$1$0$-Inf$Inf$#LKA_action_indication$0$3$2$2$1$0$1$0$-Inf$Inf$#TSR_Vision_Only_Sign_Type$48$8$2$2$1$0$1$0$-Inf$Inf$#Vehicle_Lane_Display$8$4$2$2$1$0$1$0$-Inf$Inf$#  NSignals=15  StartBits=str2num('[int32(24);int32(12);int32(18);int32(28);int32(40);int32(43);int32(32);int32(16);int32(3);int32(19);int32(5);int32(21);int32(0);int32(48);int32(8)]')  SignalSizes=str2num('[int32(4);int32(4);int32(1);int32(3);int32(3);int32(3);int32(5);int32(2);int32(2);int32(2);int32(2);int32(1);int32(3);int32(8);int32(4)]')  ByteOrders=str2num('[int32(2);int32(2);int32(2);int32(2);int32(2);int32(2);int32(2);int32(2);int32(2);int32(2);int32(2);int32(2);int32(2);int32(2);int32(2)]')  DataTypes=str2num('[int32(2);int32(2);int32(2);int32(2);int32(2);int32(2);int32(1);int32(2);int32(2);int32(2);int32(2);int32(2);int32(2);int32(2);int32(2)]')  MultiplexTypes=str2num('[int32(1);int32(1);int32(1);int32(1);int32(1);int32(1);int32(1);int32(1);int32(1);int32(1);int32(1);int32(1);int32(1);int32(1);int32(1)]')  MultiplexValues=str2num('[double(0);double(0);double(0);double(0);double(0);double(0);double(0);double(0);double(0);double(0);double(0);double(0);double(0);double(0);double(0)]')  Factors=str2num('[double(1);double(1);double(1);double(1);double(1);double(1);double(1);double(1);double(1);double(1);double(1);double(1);double(1);double(1);double(1)]')  Offsets=str2num('[double(0);double(0);double(0);double(0);double(0);double(0);double(0);double(0);double(0);double(0);double(0);double(0);double(0);double(0);double(0)]')  Minimums=str2num('[double(-Inf);double(-Inf);double(-Inf);double(-Inf);double(-Inf);double(-Inf);double(0);double(-Inf);double(-Inf);double(-Inf);double(-Inf);double(-Inf);double(-Inf);double(-Inf);double(-Inf)]')  Maximums=str2num('[double(Inf);double(Inf);double(Inf);double(Inf);double(Inf);double(Inf);double(31);double(Inf);double(Inf);double(Inf);double(Inf);double(Inf);double(Inf);double(Inf);double(Inf)]')  Remote=off  ApplyMinMax=off  BusOutput=off
      settings: SourceProductName=Simulink Real-Time  SourceProductBaseCode=XP  DataFormat=CANdb specified signals
  CAN Pack2 : canmsglib/CAN Pack  CANdbFile=D:\ADAS ECU-PSA1 CAN_for_HIL_20190729_10ms.dbc  MsgList=ADAS_3F2_PSA1  MsgName=ADAS_3F2_PSA1  MsgIDType=Standard (11-bit identifier)  MsgIdentifier=1010  MsgLength=8  SignalInfo=ABS_ESP_power_cut_request2$1$1$2$2$1$0$1$0$-Inf$Inf$#ASR_connection_dis_demand2$23$1$2$2$1$0$1$0$-Inf$Inf$#Coefficient_toregulate_EPS$41$7$2$2$1$0$1.000000e-02$0$0$1$#Column_angle_setpoint3F2$58$14$2$1$1$0$1.000000e-01$0$-780$780$#Dead_man_dedicated_push_button2$56$2$2$2$1$0$1$0$-Inf$Inf$#EASYMOVE_powercut_request3F2$3$1$2$2$1$0$1$0$-Inf$Inf$#General_state_of_LKA_function3F2$34$3$2$2$1$0$1$0$-Inf$Inf$#Permit_to_know_if_LKA_or_LPA3F2$40$1$2$2$1$0$1$0$-Inf$Inf$#Power_steering_power_cut3F2$2$1$2$2$1$0$1$0$-Inf$Inf$#Trailer_Present3F2$7$1$2$2$1$0$1$0$-Inf$Inf$#bits_compute_process_counter$8$4$2$2$1$0$1$0$-Inf$Inf$#checksum$12$4$2$2$1$0$1$0$0$15$#  NSignals=12  StartBits=str2num('[int32(1);int32(23);int32(41);int32(58);int32(56);int32(3);int32(34);int32(40);int32(2);int32(7);int32(8);int32(12)]')  SignalSizes=str2num('[int32(1);int32(1);int32(7);int32(14);int32(2);int32(1);int32(3);int32(1);int32(1);int32(1);int32(4);int32(4)]')  ByteOrders=str2num('[int32(2);int32(2);int32(2);int32(2);int32(2);int32(2);int32(2);int32(2);int32(2);int32(2);int32(2);int32(2)]')  DataTypes=str2num('[int32(2);int32(2);int32(2);int32(1);int32(2);int32(2);int32(2);int32(2);int32(2);int32(2);int32(2);int32(2)]')  MultiplexTypes=str2num('[int32(1);int32(1);int32(1);int32(1);int32(1);int32(1);int32(1);int32(1);int32(1);int32(1);int32(1);int32(1)]')  MultiplexValues=str2num('[double(0);double(0);double(0);double(0);double(0);double(0);double(0);double(0);double(0);double(0);double(0);double(0)]')  Factors=str2num('[double(1);double(1);double(1.000000e-02);double(1.000000e-01);double(1);double(1);double(1);double(1);double(1);double(1);double(1);double(1)]')  Offsets=str2num('[double(0);double(0);double(0);double(0);double(0);double(0);double(0);double(0);double(0);double(0);double(0);double(0)]')  Minimums=str2num('[double(-Inf);double(-Inf);double(0);double(-780);double(-Inf);double(-Inf);double(-Inf);double(-Inf);double(-Inf);double(-Inf);double(-Inf);double(0)]')  Maximums=str2num('[double(Inf);double(Inf);double(1);double(780);double(Inf);double(Inf);double(Inf);double(Inf);double(Inf);double(Inf);double(Inf);double(15)]')  Remote=off  ApplyMinMax=off  BusOutput=off
      settings: SourceProductName=Simulink Real-Time  SourceProductBaseCode=XP  DataFormat=CANdb specified signals
  CAN Send : S-Function  FunctionName=CAN_Send_P  Parameters=uint8(CAN_Port-1),uint8(CAN_Priority-1),uint8(S_overflow_flag),uint8(S_timestamp),double(sampletime)  SFunctionDeploymentMode=off  EnableBusSupport=off  mask{CAN_Port=CAN_1, CAN_Priority=3, S_overflow_flag=off, S_timestamp=off, sampletime=0.05}
      mask prompts: CAN_Port "CAN Port:"; CAN_Priority "Priority:"; S_overflow_flag "Send overflow flag"; S_timestamp "Send time stamp"
      mask init:
      | maskdisplay = cansendicon(CAN_Port,CAN_Priority,S_overflow_flag,S_timestamp);
      | set_param(gcb, 'MaskDisplay', maskdisplay);
      mask TypeOptions CAN_Port: CAN_0 | CAN_1 | CAN_2 | CAN_3
      mask TypeOptions CAN_Priority: 0 | 1 | 2 | 3 | 4 | 5 | 6 | 7
      mask Display: color('blue');text(0.98,0.9,'MPC5675K','horizontalAlignment','right');color('black');text(0.5,0.6,'FlexCAN_1 Send','horizontalAlignment','center');text(0.5,0.35,'Priority:3','horizontalAlignment','center');port_label('input',1,'CAN_Msg');
  CAN Send1 : S-Function  FunctionName=CAN_Send_P  Parameters=uint8(CAN_Port-1),uint8(CAN_Priority-1),uint8(S_overflow_flag),uint8(S_timestamp),double(sampletime)  SFunctionDeploymentMode=off  EnableBusSupport=off  mask{CAN_Port=CAN_1, CAN_Priority=3, S_overflow_flag=off, S_timestamp=off, sampletime=0.05}
      mask prompts: CAN_Port "CAN Port:"; CAN_Priority "Priority:"; S_overflow_flag "Send overflow flag"; S_timestamp "Send time stamp"
      mask init:
      | maskdisplay = cansendicon(CAN_Port,CAN_Priority,S_overflow_flag,S_timestamp);
      | set_param(gcb, 'MaskDisplay', maskdisplay);
      mask TypeOptions CAN_Port: CAN_0 | CAN_1 | CAN_2 | CAN_3
      mask TypeOptions CAN_Priority: 0 | 1 | 2 | 3 | 4 | 5 | 6 | 7
      mask Display: color('blue');text(0.98,0.9,'MPC5675K','horizontalAlignment','right');color('black');text(0.5,0.6,'FlexCAN_1 Send','horizontalAlignment','center');text(0.5,0.35,'Priority:3','horizontalAlignment','center');port_label('input',1,'CAN_Msg');
  CAN Send2 : S-Function  FunctionName=CAN_Send_P  Parameters=uint8(CAN_Port-1),uint8(CAN_Priority-1),uint8(S_overflow_flag),uint8(S_timestamp),double(sampletime)  SFunctionDeploymentMode=off  EnableBusSupport=off  mask{CAN_Port=CAN_0, CAN_Priority=3, S_overflow_flag=off, S_timestamp=off, sampletime=0.05}
      mask prompts: CAN_Port "CAN Port:"; CAN_Priority "Priority:"; S_overflow_flag "Send overflow flag"; S_timestamp "Send time stamp"
      mask init:
      | maskdisplay = cansendicon(CAN_Port,CAN_Priority,S_overflow_flag,S_timestamp);
      | set_param(gcb, 'MaskDisplay', maskdisplay);
      mask TypeOptions CAN_Port: CAN_0 | CAN_1 | CAN_2 | CAN_3
      mask TypeOptions CAN_Priority: 0 | 1 | 2 | 3 | 4 | 5 | 6 | 7
      mask Display: color('blue');text(0.98,0.9,'MPC5675K','horizontalAlignment','right');color('black');text(0.5,0.6,'FlexCAN_0 Send','horizontalAlignment','center');text(0.5,0.35,'Priority:3','horizontalAlignment','center');port_label('input',1,'CAN_Msg');
  CAN Send3 : S-Function  FunctionName=CAN_Send_P  Parameters=uint8(CAN_Port-1),uint8(CAN_Priority-1),uint8(S_overflow_flag),uint8(S_timestamp),double(sampletime)  SFunctionDeploymentMode=off  EnableBusSupport=off  mask{CAN_Port=CAN_0, CAN_Priority=3, S_overflow_flag=off, S_timestamp=off, sampletime=0.05}
      mask prompts: CAN_Port "CAN Port:"; CAN_Priority "Priority:"; S_overflow_flag "Send overflow flag"; S_timestamp "Send time stamp"
      mask init:
      | maskdisplay = cansendicon(CAN_Port,CAN_Priority,S_overflow_flag,S_timestamp);
      | set_param(gcb, 'MaskDisplay', maskdisplay);
      mask TypeOptions CAN_Port: CAN_0 | CAN_1 | CAN_2 | CAN_3
      mask TypeOptions CAN_Priority: 0 | 1 | 2 | 3 | 4 | 5 | 6 | 7
      mask Display: color('blue');text(0.98,0.9,'MPC5675K','horizontalAlignment','right');color('black');text(0.5,0.6,'FlexCAN_0 Send','horizontalAlignment','center');text(0.5,0.35,'Priority:3','horizontalAlignment','center');port_label('input',1,'CAN_Msg');
  D53_EPS_Control_LKA : Subsystem
  D53_HMI_Control_LKA : Subsystem
  Data Type Conversion{1..22,27..31} (27 alike) : DataTypeConversion  OutDataTypeStr=single
  Rate Transition{1..12,14..28} (27 alike) : RateTransition  Deterministic=off  OutPortSampleTime=0.05
  Rate Transition41 : RateTransition  Deterministic=off  OutPortSampleTime=0.01
  tag scope: LKA_CAL_SWA_CMD=global
  wires:
  DACOut_bsLLState/1 -> Bus Selector2/1
  Data Type Conversion12/1 -> CAN Pack2/12
  D53_EPS_Control_LKA/12(CHKSUM_TRME) -> Rate Transition11/1
  Rate Transition7/1 -> Data Type Conversion3/1
  D53_EPS_Control_LKA/1(DMD_DELEST_ABS_ESP) -> Rate Transition7/1
  D53_EPS_Control_LKA/11(CPT_PROCESS) -> Rate Transition10/1
  Data Type Conversion3/1 -> CAN Pack2/1
  Data Type Conversion10/1 -> CAN Pack2/11
  Rate Transition11/1 -> Data Type Conversion12/1
  Rate Transition10/1 -> Data Type Conversion10/1
  Rate Transition1/1 -> Data Type Conversion1/1
  Data Type Conversion6/1 -> CAN Pack2/7
  Rate Transition9/1 -> Data Type Conversion9/1
  Rate Transition4/1 -> Data Type Conversion5/1
  D53_EPS_Control_LKA/3(LKA_TRQ_FACT_REQ) -> Rate Transition2/1
  Rate Transition5/1 -> Data Type Conversion6/1
  Data Type Conversion4/1 -> Rate Transition41/1, CAN Pack2/4
  Rate Transition2/1 -> Data Type Conversion2/1
  Rate Transition3/1 -> Data Type Conversion4/1
  D53_EPS_Control_LKA/7(LKA_STATE) -> Rate Transition5/1
  Data Type Conversion9/1 -> CAN Pack2/10
  D53_EPS_Control_LKA/10(TRAILER_DETECTION) -> Rate Transition9/1
  D53_EPS_Control_LKA/9(DMD_DELEST_DA) -> Rate Transition12/1
  Data Type Conversion5/1 -> CAN Pack2/6
  D53_EPS_Control_LKA/5(ACPK_VAL_REQUEST_BSI) -> Rate Transition8/1
  Rate Transition6/1 -> Data Type Conversion8/1
  Rate Transition8/1 -> Data Type Conversion7/1
  D53_EPS_Control_LKA/8(LXA_ACTIVATION) -> Rate Transition6/1
  Data Type Conversion8/1 -> CAN Pack2/8
  D53_EPS_Control_LKA/6(DMD_DELEST_EASYMOVE) -> Rate Transition4/1
  D53_EPS_Control_LKA/2(REQ_DECON_ASR) -> Rate Transition1/1
  Data Type Conversion1/1 -> CAN Pack2/2
  D53_EPS_Control_LKA/4(COLUMN_ANGLE_SETPOINT) -> Rate Transition3/1
  Data Type Conversion7/1 -> CAN Pack2/5
  CAN Pack2/1 -> CAN Send2/1, CAN Send/1
  Data Type Conversion11/1 -> CAN Pack2/9
  Rate Transition12/1 -> Data Type Conversion11/1
  Data Type Conversion2/1 -> CAN Pack2/3
  Data Type Conversion18/1 -> CAN Pack1/1
  Rate Transition23/1 -> Data Type Conversion18/1
  D53_HMI_Control_LKA/1(ECU_operating_phase) -> Rate Transition23/1
  Rate Transition41/1 -> [LKA_CAL_SWA_CMD]
  CAN Pack1/1 -> CAN Send3/1, CAN Send1/1
  Data Type Conversion13/1 -> CAN Pack1/2
  Rate Transition14/1 -> Data Type Conversion13/1
  D53_HMI_Control_LKA/2(HMI_Popup_Status) -> Rate Transition14/1
  Data Type Conversion14/1 -> CAN Pack1/3
  Rate Transition15/1 -> Data Type Conversion14/1
  D53_HMI_Control_LKA/3(Hands_off_warning) -> Rate Transition15/1
  Data Type Conversion15/1 -> CAN Pack1/4
  Rate Transition16/1 -> Data Type Conversion15/1
  D53_HMI_Control_LKA/4(ISA_Popup_text) -> Rate Transition16/1
  Data Type Conversion16/1 -> CAN Pack1/5
  Rate Transition17/1 -> Data Type Conversion16/1
  D53_HMI_Control_LKA/5(ISA_Sign_Type) -> Rate Transition17/1
  Data Type Conversion22/1 -> CAN Pack1/6
  Rate Transition22/1 -> Data Type Conversion22/1
  D53_HMI_Control_LKA/6(ISA_Status) -> Rate Transition22/1
  Data Type Conversion17/1 -> CAN Pack1/7
  Rate Transition18/1 -> Data Type Conversion17/1
  D53_HMI_Control_LKA/7(ISA_Value) -> Rate Transition18/1
  Data Type Conversion19/1 -> CAN Pack1/8
  Rate Transition19/1 -> Data Type Conversion19/1
  D53_HMI_Control_LKA/8(LDW_Flag) -> Rate Transition19/1
  Data Type Conversion20/1 -> CAN Pack1/9
  Rate Transition20/1 -> Data Type Conversion20/1
  D53_HMI_Control_LKA/9(LDW_Status_Display) -> Rate Transition20/1
  Data Type Conversion21/1 -> CAN Pack1/10
  Rate Transition21/1 -> Data Type Conversion21/1
  D53_HMI_Control_LKA/10(LKA_Mode_from_Camera) -> Rate Transition21/1
  Data Type Conversion31/1 -> CAN Pack1/11
  Rate Transition28/1 -> Data Type Conversion31/1
  D53_HMI_Control_LKA/11(LKA_Status_Display) -> Rate Transition28/1
  Data Type Conversion27/1 -> CAN Pack1/12
  Rate Transition24/1 -> Data Type Conversion27/1
  D53_HMI_Control_LKA/12(LKA_Switch_State) -> Rate Transition24/1
  Data Type Conversion28/1 -> CAN Pack1/13
  Rate Transition25/1 -> Data Type Conversion28/1
  D53_HMI_Control_LKA/13(LKA_action_indication) -> Rate Transition25/1
  Data Type Conversion29/1 -> CAN Pack1/14
  Rate Transition26/1 -> Data Type Conversion29/1
  D53_HMI_Control_LKA/14(TSR_Vision_Only_Sign_Type) -> Rate Transition26/1
  Data Type Conversion30/1 -> CAN Pack1/15
  Rate Transition27/1 -> Data Type Conversion30/1
  D53_HMI_Control_LKA/15(Vehicle_Lane_Display) -> Rate Transition27/1
  Bus Selector2/1 -> D53_EPS_Control_LKA/4(COLUMN_ANGLE_SETPOINT_in)  "<LMS_phiSWACmd>"
  Bus Selector2/2 -> D53_EPS_Control_LKA/1(LKA_STATE_in)  "<EPS_State_Ctl>"
  Bus Selector2/3 -> D53_EPS_Control_LKA/3(LKA_TRQ_FACT_REQ_in)  "<Coefficient_toregulate_EPS>"
  Bus Selector2/4 -> D53_EPS_Control_LKA/2(LXA_ACTIVATION_in)  "<Permit_to_know_if_LKA_or_LPA3F2>"
  Bus Selector2/10 -> ?  "<LKA_Switch_State>"
  Bus Selector2/13 -> ?  "<LKA_Mode_from_Camera>"
  Bus Selector2/14 -> ?  "<TJA_HMI_Txt_Disp>"
  Bus Selector2/15 -> ?  "<TJA_status_icon>"
  Bus Selector2/11 -> Bus Creator2/5  "<Hands_off_warning>"
  Bus Selector2/7 -> Bus Creator2/6  "<LKA_action_indication>"
  Bus Creator2/1 -> D53_HMI_Control_LKA/1(LL_bsLLHMI)
  Bus Selector2/8 -> Bus Creator2/3  "<LKA_Status_Display>"
  Bus Selector2/6 -> Bus Creator2/2  "<LDW_Status_Display>"
  Bus Selector2/5 -> Bus Creator2/4  "<LDW_Flag>"
  Bus Selector2/12 -> Bus Creator2/1  "<Vehicle_Lane_Display>"
  Bus Selector2/9 -> Bus Creator2/7  "<HMI_Popup_Status>"

== system D53_LKAS_JLU_20200908_1055/Resource Initialization ==
  CAN Setup : Subsystem  mask(MPC5675K FlexCAN Setup){Device_Index=General Control Unit, CAN0_En=on, CAN0_Baudrate=500 kbps, CAN1_En=on, CAN1_Baudrate=500 kbps, CAN2_En=on, CAN2_Baudrate=500 kbps, CAN3_En=on, CAN3_Baudrate=500 kbps}
      mask prompts: Device_Index "Device"; CAN0_En "Enable FlexCAN_0"; CAN0_Baudrate "CAN_0 Baud Rate"; CAN1_En "Enable FlexCAN_1"; CAN1_Baudrate "CAN_1 Baud Rate"; CAN2_En "Enable FlexCAN_2"; CAN2_Baudrate "CAN_2 Baud Rate"; CAN3_En "Enable FlexCAN_3"; CAN3_Baudrate "CAN_3 Baud Rate"
      mask help: Assign FlexCAN modules to be used and baudrate of the selected modules.
      mask TypeOptions Device_Index: General Control Unit | Ethernet-CAN Device
      mask Callback Device_Index: CAN_en();
      mask Callback CAN0_En: CAN_en();
      mask TypeOptions CAN0_Baudrate: 125 kbps | 250 kbps | 500 kbps
      mask Callback CAN1_En: CAN_en();
      mask TypeOptions CAN1_Baudrate: 125 kbps | 250 kbps | 500 kbps
      mask Callback CAN2_En: CAN_en();
      mask TypeOptions CAN2_Baudrate: 125 kbps | 250 kbps | 500 kbps
      mask Callback CAN3_En: CAN_en();
      mask TypeOptions CAN3_Baudrate: 125 kbps | 250 kbps | 500 kbps
      mask Display: color('blue');text(0.98,0.9,'MPC5675K','horizontalAlignment','right');color('black');text(0.5,0.5,'FlexCAN Setup','horizontalAlignment','center');
  DI : Subsystem  Priority=3
  DO : Subsystem  Priority=3
  JLUVCDC ECU Master : S-Function  FunctionName=ECU_Master  Parameters=uint8(ECU_Type)  SFunctionDeploymentMode=off  EnableBusSupport=off  mask(JLUVCDC ECU Master){ECU_Type=JLUVCDC_ECU_ET4CAN_01}
      mask prompts: ECU_Type "ECU Type:"
      mask help: This block defines the ECU type for which codes are generated, also claims that the property of JLUVCDC target blocks belongs to JLUVCDC.
      mask init:
      | maskdisplay = ECUMasterIcon(ECU_Type);
      | set_param(gcb, 'MaskDisplay', maskdisplay);
      mask TypeOptions ECU_Type: JLUVCDC_ECU_GESC_01 | JLUVCDC_ECU_GMCU_01 | JLUVCDC_ECU_GVCU_01 | JLUVCDC_ECU_ET4CAN_01 | JLUVCDC_ECU_VDCU_01
      mask Display: color('blue');text(0.98,0.9,'MPC5675K','horizontalAlignment','right');color('black');text(0.5,0.5,'JLUVCDC_ECU_ET4CAN_01','horizontalAlignment','center');
  SPI : Subsystem  Priority=2

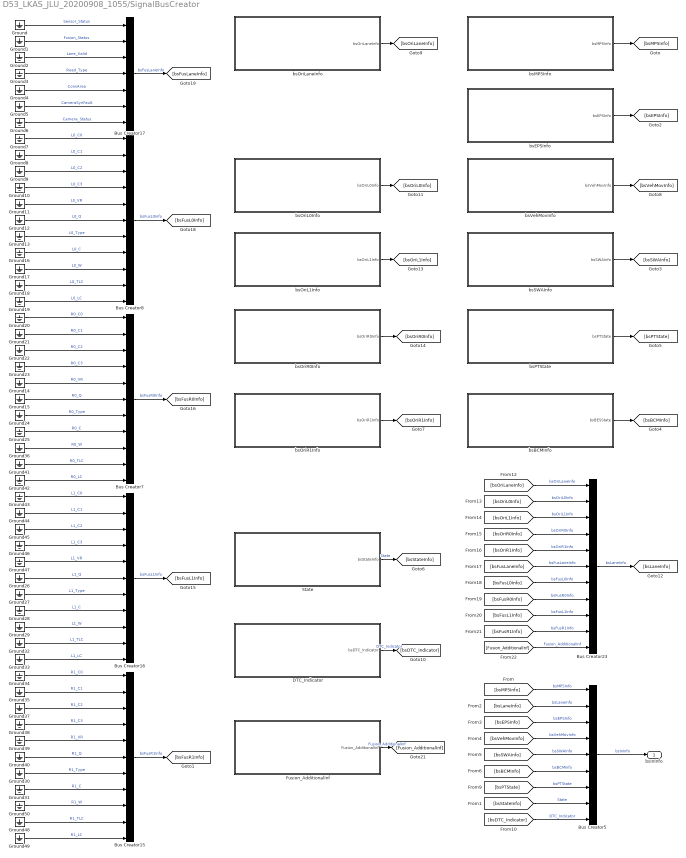
== system D53_LKAS_JLU_20200908_1055/SignalBusCreator ==
  Bus Creator{7..8,15..16,23} (5 alike) : BusCreator  Inputs=11
  Bus Creator17 : BusCreator  Inputs=7
  Bus Creator5 : BusCreator  Inputs=9
  DTC_Indicator : Subsystem
  Fusion_AdditionalInf : Subsystem
  Ground{,1..50} (51 alike) : Ground
  State : Subsystem
  bsBCMInfo : Subsystem
  bsEPSInfo : Subsystem
  bsMP5Info : Subsystem
  bsOriL0Info : Subsystem
  bsOriL1Info : Subsystem
  bsOriLaneInfo : Subsystem
  bsOriR0Info : Subsystem
  bsOriR1Info : Subsystem
  bsPTState : Subsystem
  bsSWAInfo : Subsystem
  bsVehMovInfo : Subsystem
  bsInInfo : Outport
  wires:
  bsOriL1Info/1(bsOriL1Info) -> [bsOriL1Info]
  Ground31/1 -> Bus Creator15/8  "R1_C"
  Ground38/1 -> Bus Creator15/4  "R1_C3"
  Ground30/1 -> Bus Creator15/7  "R1_Type"
  Ground29/1 -> Bus Creator16/9  "L1_W"
  Ground13/1 -> Bus Creator8/7  "L0_Type"
  Ground40/1 -> Bus Creator15/6  "R1_Q"
  Ground12/1 -> Bus Creator8/6  "L0_Q"
  Ground9/1 -> Bus Creator8/3  "L0_C2"
  Ground10/1 -> Bus Creator8/4  "L0_C3"
  [bsSWAInfo] -> Bus Creator5/5  "bsSWAInfo"
  Ground25/1 -> Bus Creator7/8  "R0_C"
  Ground23/1 -> Bus Creator7/4  "R0_C3"
  Ground27/1 -> Bus Creator16/7  "L1_Type"
  Ground28/1 -> Bus Creator16/8  "L1_C"
  Ground44/1 -> Bus Creator16/2  "L1_C1"
  Ground36/1 -> Bus Creator7/9  "R0_W"
  Ground26/1 -> Bus Creator16/6  "L1_Q"
  Ground35/1 -> Bus Creator15/2  "R1_C1"
  Ground1/1 -> Bus Creator17/2  "Fusion_Status"
  Ground24/1 -> Bus Creator7/7  "R0_Type"
  Ground41/1 -> Bus Creator7/10  "R0_TLC"
  Ground21/1 -> Bus Creator7/2  "R0_C1"
  Ground22/1 -> Bus Creator7/3  "R0_C2"
  Ground3/1 -> Bus Creator17/4  "Road_Type"
  Ground34/1 -> Bus Creator15/1  "R1_C0"
  Ground/1 -> Bus Creator17/1  "Sensor_Status"
  Ground47/1 -> Bus Creator16/5  "L1_VR"
  Ground15/1 -> Bus Creator7/6  "R0_Q"
  State/1(bsStateInfo) -> [bsStateInfo]  "State"
  Ground46/1 -> Bus Creator16/4  "L1_C3"
  Ground42/1 -> Bus Creator7/11  "R0_LC"
  Ground20/1 -> Bus Creator7/1  "R0_C0"
  Ground7/1 -> Bus Creator8/1  "L0_C0"
  Ground19/1 -> Bus Creator8/11  "L0_LC"
  Ground8/1 -> Bus Creator8/2  "L0_C1"
  Ground4/1 -> Bus Creator17/5  "ConsArea"
  Ground18/1 -> Bus Creator8/10  "L0_TLC"
  Bus Creator23/1 -> [bsLaneInfo]  "bsLaneInfo"
  Ground16/1 -> Bus Creator8/8  "L0_C"
  Ground6/1 -> Bus Creator17/7  "Camera_Status"
  Ground2/1 -> Bus Creator17/3  "Lane_Valid"
  Bus Creator8/1 -> [bsFusL0Info]  "bsFusL0Info"
  [bsFusR1Info] -> Bus Creator23/10  "bsFusR1Info"
  [Fusion_AdditionalInf] -> Bus Creator23/11  "Fusion_AdditionalInf"
  Ground14/1 -> Bus Creator7/5  "R0_VR"
  [bsFusL0Info] -> Bus Creator23/7  "bsFusL0Info"
  DTC_Indicator/1(bsDTC_Indicator) -> [bsDTC_Indicator]  "DTC_Indicator"
  [bsOriL1Info] -> Bus Creator23/3  "bsOriL1Info"
  [bsStateInfo] -> Bus Creator5/8  "State"
  Ground45/1 -> Bus Creator16/3  "L1_C2"
  Ground32/1 -> Bus Creator16/10  "L1_TLC"
  Bus Creator15/1 -> [bsFusR1Info]  "bsFusR1Info"
  Bus Creator7/1 -> [bsFusR0Info]  "bsFusR0Info"
  Ground37/1 -> Bus Creator15/3  "R1_C2"
  [bsOriL0Info] -> Bus Creator23/2  "bsOriL0Info"
  Bus Creator17/1 -> [bsFusLaneInfo]  "bsFusLaneInfo"
  [bsFusL1Info] -> Bus Creator23/9  "bsFusL1Info"
  [bsMP5Info] -> Bus Creator5/1  "bsMP5Info"
  Bus Creator16/1 -> [bsFusL1Info]  "bsFusL1Info"
  Ground11/1 -> Bus Creator8/5  "L0_VR"
  [bsOriR0Info] -> Bus Creator23/4  "bsOriR0Info"
  [bsOriLaneInfo] -> Bus Creator23/1  "bsOriLaneInfo"
  [bsLaneInfo] -> Bus Creator5/2  "bsLaneInfo"
  [bsFusR0Info] -> Bus Creator23/8  "bsFusR0Info"
  Bus Creator5/1 -> bsInInfo/1  "bsInInfo"
  [bsVehMovInfo] -> Bus Creator5/4  "bsVehMovInfo"
  [bsEPSInfo] -> Bus Creator5/3  "bsEPSInfo"
  Ground43/1 -> Bus Creator16/1  "L1_C0"
  Fusion_AdditionalInf/1(Fusion_AdditionalInf) -> [Fusion_AdditionalInf]  "Fusion_AdditionalInf"
  Ground33/1 -> Bus Creator16/11  "L1_LC"
  Ground17/1 -> Bus Creator8/9  "L0_W"
  Ground50/1 -> Bus Creator15/9  "R1_W"
  [bsDTC_Indicator] -> Bus Creator5/9  "DTC_Indicator"
  Ground5/1 -> Bus Creator17/6  "CameraSynFault"
  Ground49/1 -> Bus Creator15/11  "R1_LC"
  Ground39/1 -> Bus Creator15/5  "R1_VR"
  bsSWAInfo/1(bsSWAInfo) -> [bsSWAInfo]
  [bsOriR1Info] -> Bus Creator23/5  "bsOriR1Info"
  bsMP5Info/1(bsMP5Info) -> [bsMP5Info]
  [bsBCMInfo] -> Bus Creator5/6  "bsBCMInfo"
  [bsPTState] -> Bus Creator5/7  "bsPTState"
  bsOriL0Info/1(bsOriL0Info) -> [bsOriL0Info]
  bsOriR1Info/1(bsOriR1Info) -> [bsOriR1Info]
  bsOriLaneInfo/1(bsOriLaneInfo) -> [bsOriLaneInfo]
  Ground48/1 -> Bus Creator15/10  "R1_TLC"
  bsOriR0Info/1(bsOriR0Info) -> [bsOriR0Info]
  [bsFusLaneInfo] -> Bus Creator23/6  "bsFusLaneInfo"
  bsEPSInfo/1(bsEPSInfo) -> [bsEPSInfo]
  bsVehMovInfo/1(bsVehMovInfo) -> [bsVehMovInfo]
  bsPTState/1(bsPTState) -> [bsPTState]
  bsBCMInfo/1(bsBESState) -> [bsBCMInfo]

== system D53_LKAS_JLU_20200908_1055/CAN Monitor (CANMon)/Input ==
  In1 : Inport
  In2 : Inport  Port=2
  Bus Selector11 : BusSelector  OutputSignals=bsEPSInfo.EPS_LKA_State,bsEPSInfo.EPS_SW_Trq,bsSWAInfo.SW_Angle,bsSWAInfo.SW_Angle_Speed
  Bus Selector12 : BusSelector  OutputSignals=bsMP5Info.LKA_Main_Switch,bsMP5Info.LKA_Mode,bsPTState.TCU_ActualGear,bsLaneInfo.bsOriL0Info.O_L0_Q,bsLaneInfo.bsOriR0Info.O_R0_Q
  Bus Selector2 : BusSelector  OutputSignals=bsLaneInfo.bsOriL0Info.O_L0_C0,bsLaneInfo.bsOriL0Info.O_L0_C1,bsLaneInfo.bsOriL0Info.O_L0_C2,bsLaneInfo.bsOriL0Info.O_L0_TLC
  Bus Selector7 : BusSelector  OutputSignals=bsLaneInfo.bsOriR0Info.O_R0_C0,bsLaneInfo.bsOriR0Info.O_R0_C1,bsLaneInfo.bsOriR0Info.O_R0_C2,bsLaneInfo.bsOriR0Info.O_R0_TLC
  Bus Selector8 : BusSelector  OutputSignals=bsVehMovInfo.ESC_LatAcc,bsVehMovInfo.ESC_LonAcc,bsVehMovInfo.ESC_VehSpd,bsVehMovInfo.ESC_YawRate
  CAN Pack{16..19} (4 alike) : canmsglib/CAN Pack  CANdbFile=C:\Users\Administrator\Desktop\data_collect.dbc  MsgList=(none)  MsgName=c1deg  MsgIDType=Standard (11-bit identifier)  MsgIdentifier=2022  MsgLength=8  SignalInfo=EPSRx_trgSWTrq$8$16$2$2$1$0$0.01$0$-320$320$#EPSRx_stEPSCtlState$24$16$2$1$1$0$0.01$0$-320$320$#L0Range$40$16$2$1$1$0$1.000000e-002$0$-320$320$#R0Range$56$16$2$1$1$0$1.000000e-002$0$-320$320$#  NSignals=4  StartBits=str2num('[int32(8);int32(24);int32(40);int32(56)]')  SignalSizes=str2num('[int32(16);int32(16);int32(16);int32(16)]')  ByteOrders=str2num('[int32(2);int32(2);int32(2);int32(2)]')  DataTypes=str2num('[int32(2);int32(1);int32(1);int32(1)]')  MultiplexTypes=str2num('[int32(1);int32(1);int32(1);int32(1)]')  MultiplexValues=str2num('[double(0);double(0);double(0);double(0)]')  Factors=str2num('[double(0.01);double(0.01);double(1.000000e-002);double(1.000000e-002)]')  Offsets=str2num('[double(0);double(0);double(0);double(0)]')  Minimums=str2num('[double(-320);double(-320);double(-320);double(-320)]')  Maximums=str2num('[double(320);double(320);double(320);double(320)]')  Remote=off  ApplyMinMax=off  BusOutput=off
      settings: SourceProductName=Simulink Real-Time  SourceProductBaseCode=XP  DataFormat=manually specified signals
  CAN Pack20 : canmsglib/CAN Pack  CANdbFile=F:\LD\1_simulink\GateWay_20180716\dbc\camera_data_in.dbc  MsgList=(none)  MsgName=Video_Lane_Left_A  MsgIDType=Standard (11-bit identifier)  MsgIdentifier=1530  MsgLength=8  SignalInfo=C0$44$12$2$1$1$0$0.000001$0$-3$3$#C1$50$10$2$1$1$0$0.000001$0$-1$1$#C2$24$16$2$1$1$0$0.000001$0$-1$1$#C3$8$16$2$1$1$0$0.000001$0$-1$1$#Line_Type$59$3$2$2$1$0$1$0$0$7$#Message_Counter$48$2$2$2$1$0$1$0$0$3$#Quality$62$2$2$2$1$0$1$0$0$3$#  NSignals=7  StartBits=str2num('[int32(44);int32(50);int32(24);int32(8);int32(59);int32(48);int32(62)]')  SignalSizes=str2num('[int32(12);int32(10);int32(16);int32(16);int32(3);int32(2);int32(2)]')  ByteOrders=str2num('[int32(2);int32(2);int32(2);int32(2);int32(2);int32(2);int32(2)]')  DataTypes=str2num('[int32(1);int32(1);int32(1);int32(1);int32(2);int32(2);int32(2)]')  MultiplexTypes=str2num('[int32(1);int32(1);int32(1);int32(1);int32(1);int32(1);int32(1)]')  MultiplexValues=str2num('[double(0);double(0);double(0);double(0);double(0);double(0);double(0)]')  Factors=str2num('[double(0.000001);double(0.000001);double(0.000001);double(0.000001);double(1);double(1);double(1)]')  Offsets=str2num('[double(0);double(0);double(0);double(0);double(0);double(0);double(0)]')  Minimums=str2num('[double(-3);double(-1);double(-1);double(-1);double(0);double(0);double(0)]')  Maximums=str2num('[double(3);double(1);double(1);double(1);double(7);double(3);double(3)]')  Remote=off  ApplyMinMax=off  BusOutput=off
      settings: SourceProductName=Simulink Real-Time  SourceProductBaseCode=XP  DataFormat=manually specified signals
  CAN Send16 : S-Function  FunctionName=CAN_Send_P  Parameters=uint8(CAN_Port-1),uint8(CAN_Priority-1),uint8(S_overflow_flag),uint8(S_timestamp),double(sampletime)  SFunctionDeploymentMode=off  EnableBusSupport=off  mask{CAN_Port=CAN_0, CAN_Priority=3, S_overflow_flag=off, S_timestamp=off, sampletime=0.01}
      mask prompts: CAN_Port "CAN Port:"; CAN_Priority "Priority:"; S_overflow_flag "Send overflow flag"; S_timestamp "Send time stamp"
      mask init:
      | maskdisplay = cansendicon(CAN_Port,CAN_Priority,S_overflow_flag,S_timestamp);
      | set_param(gcb, 'MaskDisplay', maskdisplay);
      mask TypeOptions CAN_Port: CAN_0 | CAN_1 | CAN_2 | CAN_3
      mask TypeOptions CAN_Priority: 0 | 1 | 2 | 3 | 4 | 5 | 6 | 7
      mask Display: color('blue');text(0.98,0.9,'MPC5675K','horizontalAlignment','right');color('black');text(0.5,0.6,'FlexCAN_0 Send','horizontalAlignment','center');text(0.5,0.35,'Priority:3','horizontalAlignment','center');port_label('input',1,'CAN_Msg');
  CAN Send17 : S-Function  FunctionName=CAN_Send_P  Parameters=uint8(CAN_Port-1),uint8(CAN_Priority-1),uint8(S_overflow_flag),uint8(S_timestamp),double(sampletime)  SFunctionDeploymentMode=off  EnableBusSupport=off  mask{CAN_Port=CAN_0, CAN_Priority=3, S_overflow_flag=off, S_timestamp=off, sampletime=0.01}
      mask prompts: CAN_Port "CAN Port:"; CAN_Priority "Priority:"; S_overflow_flag "Send overflow flag"; S_timestamp "Send time stamp"
      mask init:
      | maskdisplay = cansendicon(CAN_Port,CAN_Priority,S_overflow_flag,S_timestamp);
      | set_param(gcb, 'MaskDisplay', maskdisplay);
      mask TypeOptions CAN_Port: CAN_0 | CAN_1 | CAN_2 | CAN_3
      mask TypeOptions CAN_Priority: 0 | 1 | 2 | 3 | 4 | 5 | 6 | 7
      mask Display: color('blue');text(0.98,0.9,'MPC5675K','horizontalAlignment','right');color('black');text(0.5,0.6,'FlexCAN_0 Send','horizontalAlignment','center');text(0.5,0.35,'Priority:3','horizontalAlignment','center');port_label('input',1,'CAN_Msg');
  CAN Send18 : S-Function  FunctionName=CAN_Send_P  Parameters=uint8(CAN_Port-1),uint8(CAN_Priority-1),uint8(S_overflow_flag),uint8(S_timestamp),double(sampletime)  SFunctionDeploymentMode=off  EnableBusSupport=off  mask{CAN_Port=CAN_0, CAN_Priority=3, S_overflow_flag=off, S_timestamp=off, sampletime=0.01}
      mask prompts: CAN_Port "CAN Port:"; CAN_Priority "Priority:"; S_overflow_flag "Send overflow flag"; S_timestamp "Send time stamp"
      mask init:
      | maskdisplay = cansendicon(CAN_Port,CAN_Priority,S_overflow_flag,S_timestamp);
      | set_param(gcb, 'MaskDisplay', maskdisplay);
      mask TypeOptions CAN_Port: CAN_0 | CAN_1 | CAN_2 | CAN_3
      mask TypeOptions CAN_Priority: 0 | 1 | 2 | 3 | 4 | 5 | 6 | 7
      mask Display: color('blue');text(0.98,0.9,'MPC5675K','horizontalAlignment','right');color('black');text(0.5,0.6,'FlexCAN_0 Send','horizontalAlignment','center');text(0.5,0.35,'Priority:3','horizontalAlignment','center');port_label('input',1,'CAN_Msg');
  CAN Send19 : S-Function  FunctionName=CAN_Send_P  Parameters=uint8(CAN_Port-1),uint8(CAN_Priority-1),uint8(S_overflow_flag),uint8(S_timestamp),double(sampletime)  SFunctionDeploymentMode=off  EnableBusSupport=off  mask{CAN_Port=CAN_0, CAN_Priority=3, S_overflow_flag=off, S_timestamp=off, sampletime=0.01}
      mask prompts: CAN_Port "CAN Port:"; CAN_Priority "Priority:"; S_overflow_flag "Send overflow flag"; S_timestamp "Send time stamp"
      mask init:
      | maskdisplay = cansendicon(CAN_Port,CAN_Priority,S_overflow_flag,S_timestamp);
      | set_param(gcb, 'MaskDisplay', maskdisplay);
      mask TypeOptions CAN_Port: CAN_0 | CAN_1 | CAN_2 | CAN_3
      mask TypeOptions CAN_Priority: 0 | 1 | 2 | 3 | 4 | 5 | 6 | 7
      mask Display: color('blue');text(0.98,0.9,'MPC5675K','horizontalAlignment','right');color('black');text(0.5,0.6,'FlexCAN_0 Send','horizontalAlignment','center');text(0.5,0.35,'Priority:3','horizontalAlignment','center');port_label('input',1,'CAN_Msg');
  CAN Send20 : S-Function  FunctionName=CAN_Send_P  Parameters=uint8(CAN_Port-1),uint8(CAN_Priority-1),uint8(S_overflow_flag),uint8(S_timestamp),double(sampletime)  SFunctionDeploymentMode=off  EnableBusSupport=off  mask{CAN_Port=CAN_0, CAN_Priority=3, S_overflow_flag=off, S_timestamp=off, sampletime=0.01}
      mask prompts: CAN_Port "CAN Port:"; CAN_Priority "Priority:"; S_overflow_flag "Send overflow flag"; S_timestamp "Send time stamp"
      mask init:
      | maskdisplay = cansendicon(CAN_Port,CAN_Priority,S_overflow_flag,S_timestamp);
      | set_param(gcb, 'MaskDisplay', maskdisplay);
      mask TypeOptions CAN_Port: CAN_0 | CAN_1 | CAN_2 | CAN_3
      mask TypeOptions CAN_Priority: 0 | 1 | 2 | 3 | 4 | 5 | 6 | 7
      mask Display: color('blue');text(0.98,0.9,'MPC5675K','horizontalAlignment','right');color('black');text(0.5,0.6,'FlexCAN_0 Send','horizontalAlignment','center');text(0.5,0.35,'Priority:3','horizontalAlignment','center');port_label('input',1,'CAN_Msg');
  Data Type Conversion{54..69} (16 alike) : DataTypeConversion  OutDataTypeStr=single
  Data Type Conversion{70..74} (5 alike) : DataTypeConversion  OutDataTypeStr=uint8
  wires:
  Data Type Conversion59/1 -> CAN Pack17/2
  Data Type Conversion60/1 -> CAN Pack17/3
  Bus Selector2/1 -> Data Type Conversion54/1  "<O_L0_C0>"
  Bus Selector12/1 -> Data Type Conversion70/1  "<LKA_Main_Switch>"
  CAN Pack18/1 -> CAN Send18/1
  Data Type Conversion66/1 -> CAN Pack19/1
  Data Type Conversion71/1 -> CAN Pack20/2
  [bsInInfo] -> Bus Selector7/1
  Data Type Conversion72/1 -> CAN Pack20/3
  Bus Selector12/4 -> Data Type Conversion73/1  "<O_L0_Q>"
  [bsInInfo] -> Bus Selector8/1
  Bus Selector2/2 -> Data Type Conversion55/1  "<O_L0_C1>"
  Data Type Conversion55/1 -> CAN Pack16/2
  Data Type Conversion57/1 -> CAN Pack16/4
  Bus Selector11/2 -> Data Type Conversion67/1  "<EPS_SW_Trq>"
  Bus Selector12/2 -> Data Type Conversion71/1  "<LKA_Mode>"
  Data Type Conversion61/1 -> CAN Pack17/4
  Bus Selector12/3 -> Data Type Conversion72/1  "<TCU_ActualGear>"
  In1/1 -> CAN Pack20/6
  Data Type Conversion64/1 -> CAN Pack18/3
  CAN Pack20/1 -> CAN Send20/1
  Bus Selector8/3 -> Data Type Conversion64/1  "<ESC_VehSpd>"
  Bus Selector8/4 -> Data Type Conversion65/1  "<ESC_YawRate>"
  Bus Selector7/1 -> Data Type Conversion58/1  "<O_R0_C0>"
  Bus Selector8/2 -> Data Type Conversion63/1  "<ESC_LonAcc>"
  In2/1 -> CAN Pack20/7
  Bus Selector7/2 -> Data Type Conversion59/1  "<O_R0_C1>"
  Bus Selector7/4 -> Data Type Conversion61/1  "<O_R0_TLC>"
  Bus Selector11/3 -> Data Type Conversion68/1  "<SW_Angle>"
  Bus Selector11/4 -> Data Type Conversion69/1  "<SW_Angle_Speed>"
  CAN Pack16/1 -> CAN Send16/1
  Data Type Conversion56/1 -> CAN Pack16/3
  Data Type Conversion70/1 -> CAN Pack20/1
  Bus Selector11/1 -> Data Type Conversion66/1  "<EPS_LKA_State>"
  Bus Selector2/3 -> Data Type Conversion56/1  "<O_L0_C2>"
  Bus Selector12/5 -> Data Type Conversion74/1  "<O_R0_Q>"
  Bus Selector8/1 -> Data Type Conversion62/1  "<ESC_LatAcc>"
  CAN Pack17/1 -> CAN Send17/1
  [bsInInfo] -> Bus Selector11/1
  Data Type Conversion58/1 -> CAN Pack17/1
  [bsInInfo] -> Bus Selector2/1
  Bus Selector7/3 -> Data Type Conversion60/1  "<O_R0_C2>"
  Bus Selector2/4 -> Data Type Conversion57/1  "<O_L0_TLC>"
  Data Type Conversion68/1 -> CAN Pack19/3
  Data Type Conversion54/1 -> CAN Pack16/1
  Data Type Conversion74/1 -> CAN Pack20/5
  CAN Pack19/1 -> CAN Send19/1
  [bsInInfo] -> Bus Selector12/1
  Data Type Conversion65/1 -> CAN Pack18/4
  Data Type Conversion63/1 -> CAN Pack18/2
  Data Type Conversion73/1 -> CAN Pack20/4
  Data Type Conversion67/1 -> CAN Pack19/2
  Data Type Conversion69/1 -> CAN Pack19/4
  Data Type Conversion62/1 -> CAN Pack18/1
